simulink model "Model_TranslationEngine64"  (R2022b)
settings: Solver=FixedStepDiscrete  StartTime=0.0  StopTime=5  RelTol=1e-3  EnableMultiTasking=on
InitFcn:
  | % Initialize model
  | ModelSettings=BTConfig.GetModelSettings();
  | 
  | ModelSettings.Validate();
  | 
  | ModelInit;
  | 
  | 
  | % load library data
  | GainLibrary_data;
  | % Load saved values from partition process
  | CapturedConstMask.LoadMapFromFile(bdroot)
StartFcn:
  | % make sure all the simulated RTC requests are found
  | %RTC_SIM_OBJ.ValidateREQs();
undefined symbols (not defined in the file or in its folder): AA, BPLP, Column, NumHFRefBPF, NumHFRefLPF, NumMusicChannels, Row, VolumeMuteConfig
libraries: TuneVar x925, TOP x490, FeaturePath x111, CapturedConstLib x52
(part 29 of 34)

== system Model_TranslationEngine64/ModelPreAmp/DecRate/Medusa5H1/MedusaHoligram/Medusa5H1 Part 3/On/VLS Gains Computation/VLS Gains Pax/Fade Tuning/Foward Downmix Max ==
  TOP : TOP/TOP  TriggerInit=[440 20 585 80]  TopName=ForwardDownmixMax  DataTypeOut=single  BankNumber=0  PreOverlay=false  PostOverlay=false  Role=Automatic
      settings: SourceProductName=Bose Talaria
  TranslateTrigger : TuneVar/TranslateTrigger  TriggerInit=[286 -100 324 -45]
      settings: SourceProductName=Bose Talaria
  Trivial Translation : MATLAB Function  TreatAsAtomicUnit=on
  Tune Variable : TuneVar/TuneVar  TuneName=ForwardDownmixMax  SpecifyMaxSize=off  VariableDim=1 (Row)  MaxSize=[1 1]  TunabilityNumber=1  MinValue=[0]  MaxValue=[1]  TriggerInit=[-70 25 100 75]  MaskValue=tuneStruct.ForwardDownmixMax
      settings: SourceProductName=Bose Talaria
  wires:
  Tune Variable/1 -> Trivial Translation/1(ForwardDownmixMax)  "ForwardDownmixMax"
  Trivial Translation/1(TOP) -> TOP/1
  TranslateTrigger/1 -> Trivial Translation/Trigger

== system Model_TranslationEngine64/ModelPreAmp/DecRate/Medusa5H1/MedusaHoligram/Medusa5H1 Part 3/On/VLS Gains Computation/VLS Gains Pax/SLC Tuning/Detent Level ==
  TOP : TOP/TOP  TriggerInit=[405 22 635 78]  TopName=DetentLevel  DataTypeOut=single  BankNumber=0  PreOverlay=false  PostOverlay=false  Role=Automatic
      settings: SourceProductName=Bose Talaria
  TranslateTrigger : TuneVar/TranslateTrigger  TriggerInit=[266 -100 304 -45]
      settings: SourceProductName=Bose Talaria
  Trivial Translation : MATLAB Function  TreatAsAtomicUnit=on
  Tune Variable : TuneVar/TuneVar  TuneName=DetentLevel  SpecifyMaxSize=off  VariableDim=1 (Row)  MaxSize=[1 1]  TunabilityNumber=1  MinValue=[0]  MaxValue=[1]  TriggerInit=[-110 25 105 75]  MaskValue=tuneStruct.detentGain
      settings: SourceProductName=Bose Talaria
  wires:
  Tune Variable/1 -> Trivial Translation/1(detentGain)  "DetentLevel"
  Trivial Translation/1(TOP) -> TOP/1
  TranslateTrigger/1 -> Trivial Translation/Trigger

== system Model_TranslationEngine64/ModelPreAmp/DecRate/Medusa5H1/MedusaHoligram/Medusa5H1 Part 3/On/VLS Gains Computation/VLS Gains Pax/SLC Tuning/Interpolation Method ==
  TOP : TOP/TOP  TriggerInit=[440 20 585 80]  TopName=Interpolation_Method  DataTypeOut=single  BankNumber=0  PreOverlay=false  PostOverlay=false  Role=Automatic
      settings: SourceProductName=Bose Talaria
  TranslateTrigger : TuneVar/TranslateTrigger  TriggerInit=[306 -100 344 -45]
      settings: SourceProductName=Bose Talaria
  Trivial Translation : MATLAB Function  TreatAsAtomicUnit=on
  Tune Variable : TuneVar/TuneVar  TuneName=Interpolation_Method  SpecifyMaxSize=off  VariableDim=1 (Row)  MaxSize=[1 1]  TunabilityNumber=2  MinValue=[0]  MaxValue=[1]  TriggerInit=[-40 25 130 75]  MaskValue=tuneStruct.interpolationMethod
      settings: SourceProductName=Bose Talaria
  wires:
  Tune Variable/1 -> Trivial Translation/1(interpolationMethod)  "Interpolation_Method"
  Trivial Translation/1(TOP) -> TOP/1
  TranslateTrigger/1 -> Trivial Translation/Trigger

== system Model_TranslationEngine64/ModelPreAmp/DecRate/Medusa5H1/MedusaHoligram/Medusa5H1 Part 3/On/VLS Gains Computation/VLS Gains Pax/SLC Tuning/Max Level ==
  TOP : TOP/TOP  TriggerInit=[425 22 630 78]  TopName=MaxLevel  DataTypeOut=single  BankNumber=0  PreOverlay=false  PostOverlay=false  Role=Automatic
      settings: SourceProductName=Bose Talaria
  TranslateTrigger : TuneVar/TranslateTrigger  TriggerInit=[306 -100 344 -45]
      settings: SourceProductName=Bose Talaria
  Trivial Translation : MATLAB Function  TreatAsAtomicUnit=on
  Tune Variable : TuneVar/TuneVar  TuneName=MaxLevel  SpecifyMaxSize=off  VariableDim=1 (Row)  MaxSize=[1 1]  TunabilityNumber=1  MinValue=[0]  MaxValue=[1]  TriggerInit=[-55 25 145 75]  MaskValue=tuneStruct.maxGain
      settings: SourceProductName=Bose Talaria
  wires:
  Tune Variable/1 -> Trivial Translation/1(maxGain)  "MaxLevel"
  Trivial Translation/1(TOP) -> TOP/1
  TranslateTrigger/1 -> Trivial Translation/Trigger

== system Model_TranslationEngine64/ModelPreAmp/DecRate/Medusa5H1/MedusaHoligram/Medusa5H1 Part 3/On/VLS Gains Computation/VLS Gains Pax/SLC Tuning/Min Level ==
  TOP : TOP/TOP  TriggerInit=[360 17 565 73]  TopName=MinLevel  DataTypeOut=single  BankNumber=0  PreOverlay=false  PostOverlay=false  Role=Automatic
      settings: SourceProductName=Bose Talaria
  TranslateTrigger : TuneVar/TranslateTrigger  TriggerInit=[231 -105 269 -50]
      settings: SourceProductName=Bose Talaria
  Trivial Translation : MATLAB Function  TreatAsAtomicUnit=on
  Tune Variable : TuneVar/TuneVar  TuneName=MinLevel  SpecifyMaxSize=off  VariableDim=1 (Row)  MaxSize=[1 1]  TunabilityNumber=1  MinValue=[0]  MaxValue=[1]  TriggerInit=[-120 20 65 70]  MaskValue=tuneStruct.minGain
      settings: SourceProductName=Bose Talaria
  wires:
  Tune Variable/1 -> Trivial Translation/1(minGain)  "MinLevel"
  Trivial Translation/1(TOP) -> TOP/1
  TranslateTrigger/1 -> Trivial Translation/Trigger

== system Model_TranslationEngine64/ModelPreAmp/DecRate/AudioPilot35/Audiopilot_3_5/NoiseEstimationVariant/RegularNoiseEstimation/HFNoiseEstimatorCoh/PostProcessing/HfImpulseRejection/ComputeSmoothingFactor/MinstatAlphaFactor ==
  TOP : TOP/TOP  TriggerInit=[440 20 585 80]  TopName=MinstatAlphaFactor  DataTypeOut=single  BankNumber=BankNumber  PreOverlay=PreOverlay  PostOverlay=PostOverlay  Role=Automatic
      settings: SourceProductName=Bose Talaria
  TrivialTranslation : TuneVar/TrivialTranslation  TriggerInit=[300 28 350 72]
      settings: SourceProductName=Bose Talaria
  Tune Variable : TuneVar/TuneVar  TuneName=MinstatAlphaFactor  SpecifyMaxSize=off  VariableDim=1 (Row)  MaxSize=[1 1]  TunabilityNumber=1  MinValue=MinValue  MaxValue=MaxValue  TriggerInit=[20 25 190 75]  MaskValue=MaskValue
      settings: SourceProductName=Bose Talaria
  wires:
  TrivialTranslation/1 -> TOP/1
  Tune Variable/1 -> TrivialTranslation/1  "MinstatAlphaFactor"

== system Model_TranslationEngine64/ModelPreAmp/DecRate/AudioPilot35/Audiopilot_3_5/NoiseEstimationVariant/RegularNoiseEstimation/HFNoiseEstimatorCoh/PostProcessing/HfImpulseRejection/ComputeSmoothingFactor/MinstatAlphaMin ==
  TOP : TOP/TOP  TriggerInit=[440 20 585 80]  TopName=MinstatAlphaMin  DataTypeOut=single  BankNumber=BankNumber  PreOverlay=PreOverlay  PostOverlay=PostOverlay  Role=Automatic
      settings: SourceProductName=Bose Talaria
  TrivialTranslation : TuneVar/TrivialTranslation  TriggerInit=[300 28 350 72]
      settings: SourceProductName=Bose Talaria
  Tune Variable : TuneVar/TuneVar  TuneName=MinstatAlphaMin  SpecifyMaxSize=off  VariableDim=1 (Row)  MaxSize=[1 1]  TunabilityNumber=1  MinValue=MinValue  MaxValue=MaxValue  TriggerInit=[20 25 190 75]  MaskValue=MaskValue
      settings: SourceProductName=Bose Talaria
  wires:
  TrivialTranslation/1 -> TOP/1
  Tune Variable/1 -> TrivialTranslation/1  "MinstatAlphaMin"

== system Model_TranslationEngine64/ModelPreAmp/DecRate/AudioPilot35/Audiopilot_3_5/NoiseEstimationVariant/RegularNoiseEstimation/HFNoiseEstimatorCoh/PostProcessing/HfImpulseRejection/IntermediateCalculation1 /MinstatBeta ==
  TOP : TOP/TOP  TriggerInit=[440 20 585 80]  TopName=MinstatBeta  DataTypeOut=single  BankNumber=BankNumber  PreOverlay=PreOverlay  PostOverlay=PostOverlay  Role=Automatic
      settings: SourceProductName=Bose Talaria
  TrivialTranslation : TuneVar/TrivialTranslation  TriggerInit=[300 28 350 72]
      settings: SourceProductName=Bose Talaria
  Tune Variable : TuneVar/TuneVar  TuneName=MinstatBeta  SpecifyMaxSize=off  VariableDim=1 (Row)  MaxSize=[1 1]  TunabilityNumber=1  MinValue=MinValue  MaxValue=MaxValue  TriggerInit=[20 25 190 75]  MaskValue=MaskValue
      settings: SourceProductName=Bose Talaria
  wires:
  TrivialTranslation/1 -> TOP/1
  Tune Variable/1 -> TrivialTranslation/1  "MinstatBeta"

== system Model_TranslationEngine64/ModelPreAmp/DecRate/AudioPilot35/Audiopilot_3_5/NoiseEstimationVariant/RegularNoiseEstimation/HFNoiseEstimatorCoh/PostProcessing/HfImpulseRejection/IntermediateCalculation1 /MinstatMin ==
  TOP : TOP/TOP  TriggerInit=[440 20 585 80]  TopName=MinstatMin  DataTypeOut=single  BankNumber=BankNumber  PreOverlay=PreOverlay  PostOverlay=PostOverlay  Role=Automatic
      settings: SourceProductName=Bose Talaria
  TrivialTranslation : TuneVar/TrivialTranslation  TriggerInit=[300 28 350 72]
      settings: SourceProductName=Bose Talaria
  Tune Variable : TuneVar/TuneVar  TuneName=MinstatMin  SpecifyMaxSize=off  VariableDim=1 (Row)  MaxSize=[1 1]  TunabilityNumber=1  MinValue=MinValue  MaxValue=MaxValue  TriggerInit=[20 25 190 75]  MaskValue=MaskValue
      settings: SourceProductName=Bose Talaria
  wires:
  TrivialTranslation/1 -> TOP/1
  Tune Variable/1 -> TrivialTranslation/1  "MinstatMin"

== system Model_TranslationEngine64/ModelPreAmp/DecRate/AudioPilot35/Audiopilot_3_5/NoiseEstimationVariant/RegularNoiseEstimation/HFNoiseEstimatorCoh/PostProcessing/HfImpulseRejection/MinSearch/FlatnessHighIndex ==
  TOP : TOP/TOP  TriggerInit=[440 20 585 80]  TopName=FlatnessHighIndex  DataTypeOut=single  BankNumber=BankNumber  PreOverlay=PreOverlay  PostOverlay=PostOverlay  Role=Automatic
      settings: SourceProductName=Bose Talaria
  TrivialTranslation : TuneVar/TrivialTranslation  TriggerInit=[300 28 350 72]
      settings: SourceProductName=Bose Talaria
  Tune Variable : TuneVar/TuneVar  TuneName=FlatnessHighIndex  SpecifyMaxSize=off  VariableDim=1 (Row)  MaxSize=[1 1]  TunabilityNumber=1  MinValue=MinValue  MaxValue=MaxValue  TriggerInit=[20 25 190 75]  MaskValue=MaskValue
      settings: SourceProductName=Bose Talaria
  wires:
  TrivialTranslation/1 -> TOP/1
  Tune Variable/1 -> TrivialTranslation/1  "FlatnessHighIndex"

== system Model_TranslationEngine64/ModelPreAmp/DecRate/AudioPilot35/Audiopilot_3_5/NoiseEstimationVariant/RegularNoiseEstimation/HFNoiseEstimatorCoh/PostProcessing/HfImpulseRejection/MinSearch/FlatnessLowIndex ==
  TOP : TOP/TOP  TriggerInit=[440 20 585 80]  TopName=FlatnessLowIndex  DataTypeOut=single  BankNumber=BankNumber  PreOverlay=PreOverlay  PostOverlay=PostOverlay  Role=Automatic
      settings: SourceProductName=Bose Talaria
  TrivialTranslation : TuneVar/TrivialTranslation  TriggerInit=[300 28 350 72]
      settings: SourceProductName=Bose Talaria
  Tune Variable : TuneVar/TuneVar  TuneName=FlatnessLowIndex  SpecifyMaxSize=off  VariableDim=1 (Row)  MaxSize=[1 1]  TunabilityNumber=1  MinValue=MinValue  MaxValue=MaxValue  TriggerInit=[20 25 190 75]  MaskValue=MaskValue
      settings: SourceProductName=Bose Talaria
  wires:
  TrivialTranslation/1 -> TOP/1
  Tune Variable/1 -> TrivialTranslation/1  "FlatnessLowIndex"

== system Model_TranslationEngine64/ModelPreAmp/DecRate/AudioPilot35/Audiopilot_3_5/NoiseEstimationVariant/RegularNoiseEstimation/HFNoiseEstimatorCoh/PostProcessing/HfImpulseRejection/MinSearch/FlatnessThreshold ==
  TOP : TOP/TOP  TriggerInit=[440 20 585 80]  TopName=FlatnessThresh  DataTypeOut=single  BankNumber=BankNumber  PreOverlay=PreOverlay  PostOverlay=PostOverlay  Role=Automatic
      settings: SourceProductName=Bose Talaria
  TrivialTranslation : TuneVar/TrivialTranslation  TriggerInit=[300 28 350 72]
      settings: SourceProductName=Bose Talaria
  Tune Variable : TuneVar/TuneVar  TuneName=FlatnessThresh  SpecifyMaxSize=off  VariableDim=1 (Row)  MaxSize=[1 1]  TunabilityNumber=1  MinValue=MinValue  MaxValue=MaxValue  TriggerInit=[20 25 190 75]  MaskValue=MaskValue
      settings: SourceProductName=Bose Talaria
  wires:
  TrivialTranslation/1 -> TOP/1
  Tune Variable/1 -> TrivialTranslation/1  "FlatnessThresh"

== system Model_TranslationEngine64/ModelPreAmp/DecRate/AudioPilot35/Audiopilot_3_5/NoiseEstimationVariant/RegularNoiseEstimation/HFNoiseEstimatorCoh/PostProcessing/HfImpulseRejection/MinSearch/MinSearchCoef ==
  TOP : TOP/TOP  TriggerInit=[440 20 585 80]  TopName=MinSearchCoef  DataTypeOut=single  BankNumber=BankNumber  PreOverlay=PreOverlay  PostOverlay=PostOverlay  Role=Automatic
      settings: SourceProductName=Bose Talaria
  TrivialTranslation : TuneVar/TrivialTranslation  TriggerInit=[300 28 350 72]
      settings: SourceProductName=Bose Talaria
  Tune Variable : TuneVar/TuneVar  TuneName=MinSearchCoef  SpecifyMaxSize=off  VariableDim=1 (Row)  MaxSize=[1 1]  TunabilityNumber=1  MinValue=MinValue  MaxValue=MaxValue  TriggerInit=[20 25 190 75]  MaskValue=MaskValue
      settings: SourceProductName=Bose Talaria
  wires:
  TrivialTranslation/1 -> TOP/1
  Tune Variable/1 -> TrivialTranslation/1  "MinSearchCoef"

== system Model_TranslationEngine64/ModelPreAmp/DecRate/AudioPilot35/Audiopilot_3_5/NoiseEstimationVariant/RegularNoiseEstimation/HFNoiseEstimatorCoh/PostProcessing/HfImpulseRejection/MinSearch/MinSearchMinGain ==
  TOP : TOP/TOP  TriggerInit=[440 20 585 80]  TopName=MinSearchMinGain  DataTypeOut=single  BankNumber=BankNumber  PreOverlay=PreOverlay  PostOverlay=PostOverlay  Role=Automatic
      settings: SourceProductName=Bose Talaria
  TrivialTranslation : TuneVar/TrivialTranslation  TriggerInit=[300 28 350 72]
      settings: SourceProductName=Bose Talaria
  Tune Variable : TuneVar/TuneVar  TuneName=MinSearchMinGain  SpecifyMaxSize=off  VariableDim=1 (Row)  MaxSize=[1 1]  TunabilityNumber=1  MinValue=MinValue  MaxValue=MaxValue  TriggerInit=[20 25 190 75]  MaskValue=MaskValue
      settings: SourceProductName=Bose Talaria
  wires:
  TrivialTranslation/1 -> TOP/1
  Tune Variable/1 -> TrivialTranslation/1  "MinSearchMinGain"

== system Model_TranslationEngine64/ModelPreAmp/DecRate/AudioPilot35/Audiopilot_3_5/NoiseEstimationVariant/RegularNoiseEstimation/HFNoiseEstimatorCoh/PostProcessing/HfImpulseRejection/MinSearch/SubWinLen ==
  Sec2Samples : MATLAB Function  TreatAsAtomicUnit=on
  TOP : TOP/TOP  TriggerInit=[5 25 270 75]  TopName=SubWinLenSamples  DataTypeOut=single  BankNumber=0  PreOverlay=false  PostOverlay=false  Role=Automatic
      settings: SourceProductName=Bose Talaria
  TranslateTrigger : TuneVar/TranslateTrigger  TriggerInit=[-129 -100 -91 -45]
      settings: SourceProductName=Bose Talaria
  Tune Variable : TuneVar/TuneVar  TuneName=SubWinTimeS  SpecifyMaxSize=off  VariableDim=1 (Row)  MaxSize=[1 1]  TunabilityNumber=1  MinValue=[]  MaxValue=[]  TriggerInit=[-520 25 -255 75]  MaskValue=Config.ImpRejSubWindowTimeSec
      settings: SourceProductName=Bose Talaria
  wires:
  Tune Variable/1 -> Sec2Samples/1(time)  "SubWinTimeS"
  Sec2Samples/1(samples) -> TOP/1
  TranslateTrigger/1 -> Sec2Samples/Trigger

== system Model_TranslationEngine64/ModelPreAmp/DecRate/AudioPilot35/Audiopilot_3_5/NoiseEstimationVariant/RegularNoiseEstimation/HFNoiseEstimatorCoh/PostProcessing/HfImpulseRejection/SmoothingNoiseFloor/LevelUpdateCoef ==
  TOP : TOP/TOP  TriggerInit=[440 20 585 80]  TopName=LevelUpdateCoef  DataTypeOut=single  BankNumber=BankNumber  PreOverlay=PreOverlay  PostOverlay=PostOverlay  Role=Automatic
      settings: SourceProductName=Bose Talaria
  TrivialTranslation : TuneVar/TrivialTranslation  TriggerInit=[300 28 350 72]
      settings: SourceProductName=Bose Talaria
  Tune Variable : TuneVar/TuneVar  TuneName=LevelUpdateCoef  SpecifyMaxSize=off  VariableDim=1 (Row)  MaxSize=[1 1]  TunabilityNumber=1  MinValue=MinValue  MaxValue=MaxValue  TriggerInit=[20 25 190 75]  MaskValue=MaskValue
      settings: SourceProductName=Bose Talaria
  wires:
  TrivialTranslation/1 -> TOP/1
  Tune Variable/1 -> TrivialTranslation/1  "LevelUpdateCoef"

== system Model_TranslationEngine64/ModelPreAmp/DecRate/AudioPilot35/Audiopilot_3_5/NoiseEstimationVariant/RegularNoiseEstimation/HFNoiseEstimatorCoh/PreProcessing/Anti-Aliasing Filter/InnerLink/PoolIirTunableWithReset ==
  CapturedTuneConst : CapturedConstLib/CapturedConst  TriggerInit=[-600 302 -500 338]  Role=Automatic
      settings: SourceProductName=Bose Talaria
  FeaturePath : FeaturePath/FeaturePath  FeatureName=PreprocessAntiAlias  IsGroup=off  GroupNumber=-1  IsModule=off  TriggerInit=[-750 -81 -635 26]
      settings: SourceProductName=Bose Talaria
  TOP : TOP/TOP  TriggerInit=[-145 187 5 243]  TopName=PooliirNumStages  DataTypeOut=uint32  BankNumber=0  PreOverlay=false  PostOverlay=Config.VariantObj.PostOverlayRequired  Role=Automatic
      settings: SourceProductName=Bose Talaria
  TOP1 : TOP/TOP  TriggerInit=[-140 277 10 333]  TopName=pooliirCoeffs  DataTypeOut=single  BankNumber=0  PreOverlay=false  PostOverlay=Config.VariantObj.PostOverlayRequired  Role=Automatic
      settings: SourceProductName=Bose Talaria
  TranslateTrigger : TuneVar/TranslateTrigger  TriggerInit=[-339 35 -301 90]
      settings: SourceProductName=Bose Talaria
  Translation : MATLAB Function  TreatAsAtomicUnit=on  mask{MaxNumStages=Config.MaxNumStages, VariantUint8=Config.Variant.Uint8Str}
      mask prompts: VariantUint8 "Variant"
  Tune Variable1 : TuneVar/TuneVar  TuneName=numStages  SpecifyMaxSize=off  VariableDim=1 (Row)  MaxSize=[1 1]  TunabilityNumber=1  MinValue=[]  MaxValue=[]  TriggerInit=[-750 235 -580 285]  MaskValue=Config.TuneDefaults.NumStages
      settings: SourceProductName=Bose Talaria
  Tune Variable2 : TuneVar/TuneVar  TuneName=sosCoefficients  SpecifyMaxSize=on  VariableDim=1 (Row)  MaxSize=[Config.MaxNumStages 6]  TunabilityNumber=1  MinValue=[]  MaxValue=[]  TriggerInit=[-750 175 -580 225]  MaskValue=Config.TuneDefaults.SosCoefficients
      settings: SourceProductName=Bose Talaria
  wires:
  TranslateTrigger/1 -> Translation/Trigger
  Tune Variable2/1 -> Translation/1(RawSOS)  "sosCoefficients"
  Translation/2(PoolCoeffs) -> TOP1/1
  Translation/1(PoolNumStages) -> TOP/1
  Tune Variable1/1 -> Translation/2(NumStages)  "numStages"
  CapturedTuneConst/1 -> Translation/3(NumChannels)

== system Model_TranslationEngine64/ModelPreAmp/DecRate/AudioPilot35/Audiopilot_3_5/NoiseEstimationVariant/RegularNoiseEstimation/HFNoiseEstimatorCoh/PreProcessing/Bandpass or Lowpass Filter/InnerLink/PoolIirTunableWithReset ==
  CapturedTuneConst : CapturedConstLib/CapturedConst  TriggerInit=[-600 302 -500 338]  Role=Automatic
      settings: SourceProductName=Bose Talaria
  FeaturePath : FeaturePath/FeaturePath  FeatureName=PreprocessBandpassLowpass  IsGroup=off  GroupNumber=-1  IsModule=off  TriggerInit=[-750 -81 -635 26]
      settings: SourceProductName=Bose Talaria
  TOP : TOP/TOP  TriggerInit=[-145 187 5 243]  TopName=PooliirNumStages  DataTypeOut=uint32  BankNumber=0  PreOverlay=false  PostOverlay=Config.VariantObj.PostOverlayRequired  Role=Automatic
      settings: SourceProductName=Bose Talaria
  TOP1 : TOP/TOP  TriggerInit=[-140 277 10 333]  TopName=pooliirCoeffs  DataTypeOut=single  BankNumber=0  PreOverlay=false  PostOverlay=Config.VariantObj.PostOverlayRequired  Role=Automatic
      settings: SourceProductName=Bose Talaria
  TranslateTrigger : TuneVar/TranslateTrigger  TriggerInit=[-339 35 -301 90]
      settings: SourceProductName=Bose Talaria
  Translation : MATLAB Function  TreatAsAtomicUnit=on  mask{MaxNumStages=Config.MaxNumStages, VariantUint8=Config.Variant.Uint8Str}
      mask prompts: VariantUint8 "Variant"
  Tune Variable1 : TuneVar/TuneVar  TuneName=numStages  SpecifyMaxSize=off  VariableDim=1 (Row)  MaxSize=[1 1]  TunabilityNumber=1  MinValue=[]  MaxValue=[]  TriggerInit=[-750 235 -580 285]  MaskValue=Config.TuneDefaults.NumStages
      settings: SourceProductName=Bose Talaria
  Tune Variable2 : TuneVar/TuneVar  TuneName=sosCoefficients  SpecifyMaxSize=on  VariableDim=1 (Row)  MaxSize=[Config.MaxNumStages 6]  TunabilityNumber=1  MinValue=[]  MaxValue=[]  TriggerInit=[-750 175 -580 225]  MaskValue=Config.TuneDefaults.SosCoefficients
      settings: SourceProductName=Bose Talaria
  wires:
  TranslateTrigger/1 -> Translation/Trigger
  Tune Variable2/1 -> Translation/1(RawSOS)  "sosCoefficients"
  Translation/2(PoolCoeffs) -> TOP1/1
  Translation/1(PoolNumStages) -> TOP/1
  Tune Variable1/1 -> Translation/2(NumStages)  "numStages"
  CapturedTuneConst/1 -> Translation/3(NumChannels)

== system Model_TranslationEngine64/ModelPreAmp/DecRate/AudioPilot35/Audiopilot_3_5/NoiseEstimationVariant/RegularNoiseEstimation/LFNoiseEstimatorCoh/LfPreProcess/FilterMic/InnerLink/PoolIirTunableWithReset ==
  CapturedTuneConst : CapturedConstLib/CapturedConst  TriggerInit=[-600 302 -500 338]  Role=Automatic
      settings: SourceProductName=Bose Talaria
  FeaturePath : FeaturePath/FeaturePath  FeatureName=Mic  IsGroup=off  GroupNumber=-1  IsModule=off  TriggerInit=[-750 -81 -635 26]
      settings: SourceProductName=Bose Talaria
  TOP : TOP/TOP  TriggerInit=[-145 187 5 243]  TopName=PooliirNumStages  DataTypeOut=uint32  BankNumber=0  PreOverlay=false  PostOverlay=Config.VariantObj.PostOverlayRequired  Role=Automatic
      settings: SourceProductName=Bose Talaria
  TOP1 : TOP/TOP  TriggerInit=[-140 277 10 333]  TopName=pooliirCoeffs  DataTypeOut=single  BankNumber=0  PreOverlay=false  PostOverlay=Config.VariantObj.PostOverlayRequired  Role=Automatic
      settings: SourceProductName=Bose Talaria
  TranslateTrigger : TuneVar/TranslateTrigger  TriggerInit=[-339 35 -301 90]
      settings: SourceProductName=Bose Talaria
  Translation : MATLAB Function  TreatAsAtomicUnit=on  mask{MaxNumStages=Config.MaxNumStages, VariantUint8=Config.Variant.Uint8Str}
      mask prompts: VariantUint8 "Variant"
  Tune Variable1 : TuneVar/TuneVar  TuneName=numStages  SpecifyMaxSize=off  VariableDim=1 (Row)  MaxSize=[1 1]  TunabilityNumber=1  MinValue=[]  MaxValue=[]  TriggerInit=[-750 235 -580 285]  MaskValue=Config.TuneDefaults.NumStages
      settings: SourceProductName=Bose Talaria
  Tune Variable2 : TuneVar/TuneVar  TuneName=sosCoefficients  SpecifyMaxSize=on  VariableDim=1 (Row)  MaxSize=[Config.MaxNumStages 6]  TunabilityNumber=1  MinValue=[]  MaxValue=[]  TriggerInit=[-750 175 -580 225]  MaskValue=Config.TuneDefaults.SosCoefficients
      settings: SourceProductName=Bose Talaria
  wires:
  TranslateTrigger/1 -> Translation/Trigger
  Tune Variable2/1 -> Translation/1(RawSOS)  "sosCoefficients"
  Translation/2(PoolCoeffs) -> TOP1/1
  Translation/1(PoolNumStages) -> TOP/1
  Tune Variable1/1 -> Translation/2(NumStages)  "numStages"
  CapturedTuneConst/1 -> Translation/3(NumChannels)

== system Model_TranslationEngine64/ModelPreAmp/DecRate/AudioPilot35/Audiopilot_3_5/NoiseEstimationVariant/RegularNoiseEstimation/LFNoiseEstimatorCoh/LfPreProcess/FilterRef/InnerLink/PoolIirTunableWithReset ==
  CapturedTuneConst : CapturedConstLib/CapturedConst  TriggerInit=[-600 302 -500 338]  Role=Automatic
      settings: SourceProductName=Bose Talaria
  FeaturePath : FeaturePath/FeaturePath  FeatureName=Ref  IsGroup=off  GroupNumber=-1  IsModule=off  TriggerInit=[-750 -81 -635 26]
      settings: SourceProductName=Bose Talaria
  TOP : TOP/TOP  TriggerInit=[-145 187 5 243]  TopName=PooliirNumStages  DataTypeOut=uint32  BankNumber=0  PreOverlay=false  PostOverlay=Config.VariantObj.PostOverlayRequired  Role=Automatic
      settings: SourceProductName=Bose Talaria
  TOP1 : TOP/TOP  TriggerInit=[-140 277 10 333]  TopName=pooliirCoeffs  DataTypeOut=single  BankNumber=0  PreOverlay=false  PostOverlay=Config.VariantObj.PostOverlayRequired  Role=Automatic
      settings: SourceProductName=Bose Talaria
  TranslateTrigger : TuneVar/TranslateTrigger  TriggerInit=[-339 35 -301 90]
      settings: SourceProductName=Bose Talaria
  Translation : MATLAB Function  TreatAsAtomicUnit=on  mask{MaxNumStages=Config.MaxNumStages, VariantUint8=Config.Variant.Uint8Str}
      mask prompts: VariantUint8 "Variant"
  Tune Variable1 : TuneVar/TuneVar  TuneName=numStages  SpecifyMaxSize=off  VariableDim=1 (Row)  MaxSize=[1 1]  TunabilityNumber=1  MinValue=[]  MaxValue=[]  TriggerInit=[-750 235 -580 285]  MaskValue=Config.TuneDefaults.NumStages
      settings: SourceProductName=Bose Talaria
  Tune Variable2 : TuneVar/TuneVar  TuneName=sosCoefficients  SpecifyMaxSize=on  VariableDim=1 (Row)  MaxSize=[Config.MaxNumStages 6]  TunabilityNumber=1  MinValue=[]  MaxValue=[]  TriggerInit=[-750 175 -580 225]  MaskValue=Config.TuneDefaults.SosCoefficients
      settings: SourceProductName=Bose Talaria
  wires:
  TranslateTrigger/1 -> Translation/Trigger
  Tune Variable2/1 -> Translation/1(RawSOS)  "sosCoefficients"
  Translation/2(PoolCoeffs) -> TOP1/1
  Translation/1(PoolNumStages) -> TOP/1
  Tune Variable1/1 -> Translation/2(NumStages)  "numStages"
  CapturedTuneConst/1 -> Translation/3(NumChannels)

== system Model_TranslationEngine64/ModelPreAmp/DecRate/Medusa5H1/MedusaHoligram/Medusa5H1 Part 2/Decimated-Rate FDP/Fdp/FreqDomainProcessing/CalculateAndApplyCoefficients/DeciRate/Calculate coefficients ==
  note: Rate Transition blocks are inserted after TOPs to convert their sample rate
      | to decimated rate. Initially their sample rate is inherited from the fastest one
      | of all the blocks that use it, which happen to be either inside full-rate block,
      | or the fastest sample rate in the model.
  FeaturePath : FeaturePath/FeaturePath  FeatureName=Coeffs  IsGroup=off  GroupNumber=-1  IsModule=off  TriggerInit=[-545 -1 -430 106]
      settings: SourceProductName=Bose Talaria
  StretchParamsTuning : Subsystem

== system Model_TranslationEngine64/ModelPreAmp/DecRate/Medusa5H1/MedusaHoligram/Medusa5H1 Part 2/Full-Rate FDP/Fdp/FreqDomainProcessing/CalculateAndApplyCoefficients/FullRate/Calculate coefficients ==
  FeaturePath : FeaturePath/FeaturePath  FeatureName=Coeffs  IsGroup=off  GroupNumber=-1  IsModule=off  TriggerInit=[1075 99 1190 206]
      settings: SourceProductName=Bose Talaria
  StretchParams : Subsystem

== system Model_TranslationEngine64/ModelPreAmp/DecRate/Medusa5H1/MedusaHoligram/Medusa5H1 Part 2/Decimated-Rate FDP/Fdp/FreqDomainProcessing/CalculateAndApplyCoefficients/DeciRate/Calculate coefficients/StretchParamsTuning ==
  TOP : TOP/TOP  TriggerInit=[1190 -388 1425 -332]  TopName=XpMax  DataTypeOut=single  BankNumber=0  PreOverlay=false  PostOverlay=false  Role=Automatic
      settings: SourceProductName=Bose Talaria
  TOP1 : TOP/TOP  TriggerInit=[1190 -310 1425 -250]  TopName=LokRokMaxScaleFactor  DataTypeOut=single  BankNumber=0  PreOverlay=false  PostOverlay=false  Role=Automatic
      settings: SourceProductName=Bose Talaria
  TOP2 : TOP/TOP  TriggerInit=[1195 -83 1430 -17]  TopName=ESDUpperbounddB  DataTypeOut=single  BankNumber=0  PreOverlay=false  PostOverlay=false  Role=Automatic
      settings: SourceProductName=Bose Talaria
  TOP3 : TOP/TOP  TriggerInit=[1195 0 1430 60]  TopName=ESDLowerbounddB  DataTypeOut=single  BankNumber=0  PreOverlay=false  PostOverlay=false  Role=Automatic
      settings: SourceProductName=Bose Talaria
  TOP4 : TOP/TOP  TriggerInit=[1195 80 1430 140]  TopName=ESDStepSize  DataTypeOut=single  BankNumber=0  PreOverlay=false  PostOverlay=false  Role=Automatic
      settings: SourceProductName=Bose Talaria
  TOP5 : TOP/TOP  TriggerInit=[1190 -230 1425 -170]  TopName=XpMin  DataTypeOut=single  BankNumber=0  PreOverlay=false  PostOverlay=false  Role=Automatic
      settings: SourceProductName=Bose Talaria
  TranslateTrigger : TuneVar/TranslateTrigger  TriggerInit=[1036 -460 1074 -425]
      settings: SourceProductName=Bose Talaria
  TranslateTrigger3 : TuneVar/TranslateTrigger  TriggerInit=[1041 -145 1079 -110]
      settings: SourceProductName=Bose Talaria
  Trivial Translation : MATLAB Function  TreatAsAtomicUnit=on
  Trivial Translation3 : MATLAB Function  TreatAsAtomicUnit=on
  Tune Variable1 : TuneVar/TuneVar  Description=Upper threshold on Excessive Stretch Detector (ESD) metric.  TuneName=ESDUpperbounddB  SpecifyMaxSize=off  VariableDim=1 (Row)  MaxSize=[1 1]  TunabilityNumber=1  MinValue=[]  MaxValue=[]  TriggerInit=[20 425 245 475]  MaskValue=Config.TuneDefaults.FdpCoeffsESDUpperbounddB
      settings: SourceProductName=Bose Talaria
  Tune Variable2 : TuneVar/TuneVar  Description=Lower threshold on Excessive Stretch Detector (ESD) metric.  TuneName=ESDLowerbounddB  SpecifyMaxSize=off  VariableDim=1 (Row)  MaxSize=[1 1]  TunabilityNumber=1  MinValue=[]  MaxValue=[]  TriggerInit=[20 545 240 595]  MaskValue=Config.TuneDefaults.FdpCoeffsDeciRateESDLowerbounddB
      settings: SourceProductName=Bose Talaria
  Tune Variable3 : TuneVar/TuneVar  Description=Minimum stretch factor - must be in range [0,1).  TuneName=XpMin  SpecifyMaxSize=off  VariableDim=1 (Row)  MaxSize=[1 1]  TunabilityNumber=1  MinValue=0  MaxValue=1  TriggerInit=[45 235 215 285]  MaskValue=Config.TuneDefaults.FdpCoeffsXpMin
      settings: SourceProductName=Bose Talaria
  wires:
  Tune Variable1/1 -> Trivial Translation3/1(ESDUpperbounddBIn)  "ESDUpperbounddB"
  Trivial Translation3/1(ESDUpperbounddB) -> TOP2/1
  TranslateTrigger/1 -> Trivial Translation/Trigger
  TranslateTrigger3/1 -> Trivial Translation3/Trigger
  Trivial Translation/3(XpMin) -> TOP5/1
  Trivial Translation3/2(ESDLowerbounddB) -> TOP3/1
  Trivial Translation/1(XpMax) -> TOP/1
  Tune Variable3/1 -> Trivial Translation/2(XpMinIn)  "XpMin"
  Trivial Translation/2(LokRokMaxScaleFactor) -> TOP1/1
  [deciRateXpMax] -> Trivial Translation/1(XpMaxIn)  "XpMax"
  Trivial Translation3/3(ESDStepSize) -> TOP4/1
  Tune Variable2/1 -> Trivial Translation3/2(ESDLowerbounddBIn)  "ESDLowerbounddB"

== system Model_TranslationEngine64/ModelPreAmp/DecRate/Medusa5H1/MedusaHoligram/Medusa5H1 Part 2/Full-Rate FDP/Fdp/FreqDomainProcessing/CalculateAndApplyCoefficients/FullRate/Calculate coefficients/StretchParams ==
  TOP : TOP/TOP  TriggerInit=[970 -388 1200 -332]  TopName=XpMax  DataTypeOut=single  BankNumber=0  PreOverlay=false  PostOverlay=false  Role=Automatic
      settings: SourceProductName=Bose Talaria
  TOP1 : TOP/TOP  TriggerInit=[970 -310 1205 -250]  TopName=LokRokMaxScaleFactor  DataTypeOut=single  BankNumber=0  PreOverlay=false  PostOverlay=false  Role=Automatic
      settings: SourceProductName=Bose Talaria
  TOP2 : TOP/TOP  TriggerInit=[970 -78 1205 -12]  TopName=ESDUpperbounddB  DataTypeOut=single  BankNumber=0  PreOverlay=false  PostOverlay=false  Role=Automatic
      settings: SourceProductName=Bose Talaria
  TOP3 : TOP/TOP  TriggerInit=[970 5 1205 65]  TopName=ESDLowerbounddB  DataTypeOut=single  BankNumber=0  PreOverlay=false  PostOverlay=false  Role=Automatic
      settings: SourceProductName=Bose Talaria
  TOP4 : TOP/TOP  TriggerInit=[970 85 1205 145]  TopName=ESDStepSize  DataTypeOut=single  BankNumber=0  PreOverlay=false  PostOverlay=false  Role=Automatic
      settings: SourceProductName=Bose Talaria
  TOP5 : TOP/TOP  TriggerInit=[970 -230 1205 -170]  TopName=XpMin  DataTypeOut=single  BankNumber=0  PreOverlay=false  PostOverlay=false  Role=Automatic
      settings: SourceProductName=Bose Talaria
  TranslateTrigger : TuneVar/TranslateTrigger  TriggerInit=[816 -460 854 -425]
      settings: SourceProductName=Bose Talaria
  TranslateTrigger3 : TuneVar/TranslateTrigger  TriggerInit=[816 -140 854 -105]
      settings: SourceProductName=Bose Talaria
  Trivial Translation : MATLAB Function  TreatAsAtomicUnit=on
  Trivial Translation3 : MATLAB Function  TreatAsAtomicUnit=on
  Tune Variable : TuneVar/TuneVar  Description=Maximum stretch factor - must be in range [0,1).  TuneName=XpMax  SpecifyMaxSize=off  VariableDim=1 (Row)  MaxSize=[1 1]  TunabilityNumber=1  MinValue=0  MaxValue=1  TriggerInit=[45 95 215 145]  MaskValue=Config.TuneDefaults.FdpFullRateXpMax
      settings: SourceProductName=Bose Talaria
  Tune Variable1 : TuneVar/TuneVar  Description=Upper threshold on Excessive Stretch Detector (ESD) metric.  TuneName=ESDUpperbounddB  SpecifyMaxSize=off  VariableDim=1 (Row)  MaxSize=[1 1]  TunabilityNumber=1  MinValue=[]  MaxValue=[]  TriggerInit=[20 430 235 480]  MaskValue=Config.TuneDefaults.FdpCoeffsESDUpperbounddB
      settings: SourceProductName=Bose Talaria
  Tune Variable2 : TuneVar/TuneVar  Description=Lower threshold on Excessive Stretch Detector (ESD) metric.  TuneName=ESDLowerbounddB  SpecifyMaxSize=off  VariableDim=1 (Row)  MaxSize=[1 1]  TunabilityNumber=1  MinValue=[]  MaxValue=[]  TriggerInit=[20 550 235 600]  MaskValue=Config.TuneDefaults.FdpCoeffsFullRateESDLowerbounddB
      settings: SourceProductName=Bose Talaria
  Tune Variable3 : TuneVar/TuneVar  Description=Minimum stretch factor - must be in range [0,1)  TuneName=XpMin  SpecifyMaxSize=off  VariableDim=1 (Row)  MaxSize=[1 1]  TunabilityNumber=1  MinValue=0  MaxValue=1  TriggerInit=[45 175 215 225]  MaskValue=Config.TuneDefaults.FdpCoeffsXpMin
      settings: SourceProductName=Bose Talaria
  wires:
  Tune Variable3/1 -> Trivial Translation/2(XpMinIn)  "XpMin"
  [deciRateXpMax] -> Trivial Translation/3(deciXpMaxIn)  "XpMax"
  Trivial Translation/1(XpMax) -> TOP/1
  Tune Variable2/1 -> Trivial Translation3/2(ESDLowerbounddBIn)  "ESDLowerbounddB"
  Tune Variable/1 -> Trivial Translation/1(XpMaxIn)  "XpMax"
  Trivial Translation3/2(ESDLowerbounddB) -> TOP3/1
  TranslateTrigger/1 -> Trivial Translation/Trigger
  Trivial Translation3/1(ESDUpperbounddB) -> TOP2/1
  Trivial Translation3/3(ESDStepSize) -> TOP4/1
  Trivial Translation/3(XpMin) -> TOP5/1
  TranslateTrigger3/1 -> Trivial Translation3/Trigger
  Trivial Translation/2(LokRokMaxScaleFactor) -> TOP1/1
  Tune Variable1/1 -> Trivial Translation3/1(ESDUpperbounddBIn)  "ESDUpperbounddB"

== matlab function Model_TranslationEngine64/ModelPreAmp/DecRate/Medusa5H1/MedusaHoligram/Medusa5H1 Part 3/On/VLS Gains Computation/VLS Gains Drv/SLC Tuning/Interpolation Method/Trivial Translation ==
  data: TOP output; interpolationMethod input
  events: trigger input FUNCTION_CALL_EVENT
function TOP  = fcn(interpolationMethod)
%#codegen
% Checks if the parameter satisfies dimensionality requirements
if(numel(interpolationMethod.Value) ~= 1)
   TranslateError('The parameter ''medusa_surround_db_interpolation'' must be single dimensional.'); 
end

% Checks if the parameter value follows bound requirements
if((interpolationMethod.Value ~= 0) && (interpolationMethod.Value ~= 1))
   TranslateError('The value of ''medusa_surround_db_interpolation'' must be either 0 (for linear interpolation) or 1 (for dB-linear interpolation).'); 
end

TOP = interpolationMethod.Value;

end

== matlab function Model_TranslationEngine64/ModelPreAmp/DecRate/AudioPilot35/EntertainmentLevelDetection/AudiopilotLevelDetect/AudiopilotLevelDetect/FastDecay/sec2samples ==
  data: y output; u input; FrameRate parameter
  events: trigger input FUNCTION_CALL_EVENT
function y  = fcn(u,FrameRate)
%#codegen

y = -abs(u.Value/FrameRate);

== matlab function Model_TranslationEngine64/ModelPreAmp/DecRate/Medusa5H1/MedusaHoligram/Medusa5H1 Part 3/On/VLS Gains Computation/VLS Gains Drv/SLC Tuning/Max Level/Trivial Translation ==
  data: TOP output; maxGain input; configStruct parameter
  events: trigger input FUNCTION_CALL_EVENT
function TOP  = fcn(maxGain, configStruct)
%#codegen

% Checks if the parameter satisfies dimensionality requirements
if(maxGain.Size(1) ~= configStruct.numGains)
    TranslateError('The parameter ''VLS_gains_max'' must be a %d element vector.', configStruct.numGains);
end

% Checks if the parameter values follow bound requirements
checkValues = (maxGain.Value < 0);
if(sum(sum(checkValues)))          % Results in 0 if all values in the matrix respect the bound requirements
    TranslateError('The weights in ''VLS_gains_max'' must be greater than or equal to 0.');
end

TOP = maxGain.Value;

end

== matlab function Model_TranslationEngine64/ModelPreAmp/DecRate/Medusa5H1/MedusaHoligram/Medusa5H1 Part 3/On/VLS Gains Computation/VLS Gains Drv/SLC Tuning/Min Level/Trivial Translation ==
  data: TOP output; minGain input; configStruct parameter
  events: trigger input FUNCTION_CALL_EVENT
function TOP  = fcn(minGain, configStruct)
%#codegen

% Checks if the parameter satisfies dimensionality requirements
if(minGain.Size(1) ~= configStruct.numGains)
    TranslateError('The parameter ''VLS_gains_min'' must be a %d element vector.', configStruct.numGains);
end

% Checks if the parameter values follow bound requirements
checkValues = (minGain.Value < 0);
if(sum(sum(checkValues)))          % Results in 0 if all values in the matrix respect the bound requirements
    TranslateError('The weights in ''VLS_gains_min'' must be greater than or equal to 0.');
end

TOP = minGain.Value;

end

== matlab function Model_TranslationEngine64/ModelPreAmp/DecRate/Medusa5H1/MedusaHoligram/Medusa5H1 Part 3/On/VLS Gains Computation/VLS Gains Pax/Fade Tuning/Forward Downmix Threshold/Trivial Translation ==
  data: TOP output; ForwardDownmixThreshold input
  events: trigger input FUNCTION_CALL_EVENT
function TOP  = fcn(ForwardDownmixThreshold)
%#codegen
% Checks if the parameter satisfies dimensionality requirements
if(numel(ForwardDownmixThreshold.Value) ~= 1)
   TranslateError('The parameter ''medusa_forward_downmix_threshold'' must be single dimensional.'); 
end

% Checks if the parameter value follows bound requirements
if((ForwardDownmixThreshold.Value < 0) || (ForwardDownmixThreshold.Value > 1))
   TranslateError('The value of ''medusa_forward_downmix_threshold'' must be between 0 and 1.'); 
end

TOP = ForwardDownmixThreshold.Value;

end

== matlab function Model_TranslationEngine64/ModelPreAmp/DecRate/Medusa5H1/MedusaHoligram/Medusa5H1 Part 3/On/VLS Gains Computation/VLS Gains Pax/Fade Tuning/Foward Downmix Max/Trivial Translation ==
  data: TOP output; ForwardDownmixMax input
  events: trigger input FUNCTION_CALL_EVENT
function TOP  = fcn(ForwardDownmixMax)
%#codegen
% Checks if the parameter satisfies dimensionality requirements
if(numel(ForwardDownmixMax.Value) ~= 1)
   TranslateError('The parameter ''medusa_forward_downmix_max'' must be single dimensional.'); 
end

% Checks if the parameter value follows bound requirements
if((ForwardDownmixMax.Value < 0) || (ForwardDownmixMax.Value > 1))
   TranslateError('The value of ''medusa_forward_downmix_max'' must be between 0 and 1.'); 
end

TOP = ForwardDownmixMax.Value;

end

== matlab function Model_TranslationEngine64/ModelPreAmp/DecRate/Medusa5H1/MedusaHoligram/Medusa5H1 Part 4/On/FR IIR Holigram EQ/IIR/PoolIirTunableWithReset/Translation ==
  data: RawSOS input; NumStages input; PoolNumStages output; PoolCoeffs output; MaxNumStages parameter; VariantUint8 parameter; NumChannels input
  events: trigger input FUNCTION_CALL_EVENT
function [PoolNumStages, PoolCoeffs] = pooliirTranslation(RawSOS, NumStages, MaxNumStages, VariantUint8,  NumChannels)
%#codegen

% Translation from raw SOS for pool SOS

% Some build time sanity size checking before calling the translation
if numel(NumStages.Value) ~= NumChannels
    error('Size of num stages has to match number of input channels')
end

if RawSOS.Size(2) ~= 6
    error ('Coefficient pool matrix must have 6 columns')
end

[PoolNumStages, PoolCoeffs] = poolIirTranslation(RawSOS, NumStages, MaxNumStages, VariantUint8);

% VariantStr = char(VariantUint8);
% switch (VariantStr)
%     case {"Generic","SharcPlusCore"}
%         % These variants order biquad coefficients in a compacted form
%         [PoolNumStages, PoolCoeffs] = pooliirTranslationFcn(RawSOS, NumStages, MaxNumStages);
%     case {"SharcPlusAccelGul","SharcPlusAccelGxp"}
%         % These variants order biquad coefficients for the ADI accelerator
%         [PoolNumStages, PoolCoeffs] = pooliirAccelTranslationFcn(RawSOS, NumStages, MaxNumStages);
%     case{"Hexagon"}
%         % Hexagon specific order for biquad coefficients 
%         [PoolNumStages, PoolCoeffs] = PoolIirHexagonTranslationFcn(RawSOS, NumStages, MaxNumStages);
%     case{"ArmNeonV7V8"}
%         [PoolNumStages, PoolCoeffs] = PoolIirArmNeonV7V8TranslationFcn(RawSOS, NumStages, MaxNumStages);
%     otherwise
%         % This is a build-time error, not a translation error. The
%         % selected build-time variant is not supported for translation
%         error('Invalid implementation type: [%s]', VariantStr);
% end

end

== matlab function Model_TranslationEngine64/ModelPreAmp/DecRate/Medusa5H1/MedusaHoligram/Medusa5H1 Part 4/On/DR Mix Matrix with Hybrid Holigram EQ/Tune Translations/translation ==
  data: FIRCoeffs output; FIRCoeffsIn input; FIRLengths output; FIRLengthsIn input; PaddedFIRLengthsIn input; PaddedFIRLengths output
  events: trigger input FUNCTION_CALL_EVENT
function [FIRCoeffs, FIRLengths, PaddedFIRLengths] = fcn(FIRCoeffsIn, FIRLengthsIn, PaddedFIRLengthsIn)

FIRCoeffs = FIRCoeffsIn.Value;
FIRLengths = FIRLengthsIn.Value;
PaddedFIRLengths = PaddedFIRLengthsIn.Value;

== matlab function Model_TranslationEngine64/ModelPreAmp/DecRate/Medusa5H1/MedusaHoligram/Medusa5H1 Part 4/On/Headrest Comp EQ/IIR/PoolIirTunableWithReset/Translation ==
  data: RawSOS input; NumStages input; PoolNumStages output; PoolCoeffs output; MaxNumStages parameter; VariantUint8 parameter; NumChannels input
  events: trigger input FUNCTION_CALL_EVENT
function [PoolNumStages, PoolCoeffs] = pooliirTranslation(RawSOS, NumStages, MaxNumStages, VariantUint8,  NumChannels)
%#codegen

% Translation from raw SOS for pool SOS

% Some build time sanity size checking before calling the translation
if numel(NumStages.Value) ~= NumChannels
    error('Size of num stages has to match number of input channels')
end

if RawSOS.Size(2) ~= 6
    error ('Coefficient pool matrix must have 6 columns')
end

[PoolNumStages, PoolCoeffs] = poolIirTranslation(RawSOS, NumStages, MaxNumStages, VariantUint8);

% VariantStr = char(VariantUint8);
% switch (VariantStr)
%     case {"Generic","SharcPlusCore"}
%         % These variants order biquad coefficients in a compacted form
%         [PoolNumStages, PoolCoeffs] = pooliirTranslationFcn(RawSOS, NumStages, MaxNumStages);
%     case {"SharcPlusAccelGul","SharcPlusAccelGxp"}
%         % These variants order biquad coefficients for the ADI accelerator
%         [PoolNumStages, PoolCoeffs] = pooliirAccelTranslationFcn(RawSOS, NumStages, MaxNumStages);
%     case{"Hexagon"}
%         % Hexagon specific order for biquad coefficients 
%         [PoolNumStages, PoolCoeffs] = PoolIirHexagonTranslationFcn(RawSOS, NumStages, MaxNumStages);
%     case{"ArmNeonV7V8"}
%         [PoolNumStages, PoolCoeffs] = PoolIirArmNeonV7V8TranslationFcn(RawSOS, NumStages, MaxNumStages);
%     otherwise
%         % This is a build-time error, not a translation error. The
%         % selected build-time variant is not supported for translation
%         error('Invalid implementation type: [%s]', VariantStr);
% end

end

== matlab function Model_TranslationEngine64/ModelPreAmp/DecRate/Medusa5H1/MedusaHoligram/Medusa5H1 Part 4/On/Headrest Comp EQ/translation ==
  data: FIRCoeffs output; FIRCoeffsIn input; FIRLengths output; FIRLengthsIn input; PaddedFIRLengthsIn input; PaddedFIRLengths output
  events: trigger input FUNCTION_CALL_EVENT
function [FIRCoeffs, FIRLengths, PaddedFIRLengths] = fcn(FIRCoeffsIn, FIRLengthsIn, PaddedFIRLengthsIn)

FIRCoeffs = FIRCoeffsIn.Value;
FIRLengths = FIRLengthsIn.Value;
PaddedFIRLengths = PaddedFIRLengthsIn.Value;

== matlab function Model_TranslationEngine64/ModelPreAmp/DecRate/Medusa5H1/MedusaHoligram/Medusa5H1 Part 6/Speaker Delay Tune/Output Delay Translation with Headrest/translation ==
  data: tuneNonHRDelaySamples input; tuneHRDrvDelaySamples input; tuneHRPaxDelaySamples input; tuneFREQDelaySamples input; DRDelay output; FRSpkrDelay output; DecimationFactor parameter; maxFullRateHoligramDelay parameter; maxFullRateSpeakerDelay parameter; numHeadrestComps parameter
  events: trigger input FUNCTION_CALL_EVENT
function [DRDelay, FRSpkrDelay] = fcn( tuneNonHRDelaySamples, tuneHRDrvDelaySamples, ...
    tuneHRPaxDelaySamples, tuneFREQDelaySamples, DecimationFactor, maxFullRateHoligramDelay, maxFullRateSpeakerDelay, numHeadrestComps)
%#codegen
%[Param:DecimationFactor]
%[Param:maxFullRateHoligramDelay]
%[Param:maxFullRateSpeakerDelay]
%[Param:numHeadrestComps]

nonHRDelaySamples = tuneNonHRDelaySamples.Value;
HRDrvDelaySamples = tuneHRDrvDelaySamples.Value;
HRPaxDelaySamples = tuneHRPaxDelaySamples.Value;
FREQDelaySamples = int32(tuneFREQDelaySamples.Value);

% Get delay upper bounds
maxFREQDelay = maxFullRateHoligramDelay;
maxFRSpkrDelay = maxFullRateSpeakerDelay;

% Compute delay values in samples
DEC = DecimationFactor;
% sampleRate = sampleRate;
FRHRDrvDelaySamples = round(HRDrvDelaySamples);
FRHRPaxDelaySamples = round(HRPaxDelaySamples);
FRNonHRDelaySamples = round(nonHRDelaySamples);

% Check whether speaker delays are multiple of 4, and if not round them up 
% to the nearest multiple
rem = ceil(FRNonHRDelaySamples/4)*4 - FRNonHRDelaySamples;
FRNonHRDelaySamples = int32(FRNonHRDelaySamples + rem);
DRNonHRDelaySamples = int32(FRNonHRDelaySamples/DEC);
if any(rem ~= 0)
    TranslateError('Speaker delays must be a multiple of 4.');
end

rem = ceil(FRHRDrvDelaySamples/4)*4 - FRHRDrvDelaySamples;
FRHRDrvDelaySamples = int32(FRHRDrvDelaySamples + rem);
DRHRDrvDelaySamples = int32(FRHRDrvDelaySamples/DEC);
if any(rem ~= 0)
    TranslateError('Driver headrest speaker delay must be a multiple of 4.');
end

rem = ceil(FRHRPaxDelaySamples/4)*4 - FRHRPaxDelaySamples;
FRHRPaxDelaySamples = int32(FRHRPaxDelaySamples + rem);
DRHRPaxDelaySamples = int32(FRHRPaxDelaySamples/DEC);
if any(rem ~= 0)
    TranslateError('Passenger headrest speaker delay must be a multiple of 4.');
end

% Check if delays are within bounds
checkDelay(FREQDelaySamples, maxFREQDelay, 'Medusa HFEQ delay');
checkDelay(FRHRDrvDelaySamples, maxFRSpkrDelay, 'h01/h0r delay');
checkDelay(FRHRPaxDelaySamples, maxFRSpkrDelay, 'h1l/h1r delay');
checkDelay(FRNonHRDelaySamples, maxFRSpkrDelay, 'Medusa non-headrest speaker delay');

% Assign values to TOPs
HRcomps = int32(ones(1,numHeadrestComps));
HRDrvDelay = DRHRDrvDelaySamples * HRcomps;
HRPaxDelay = DRHRPaxDelaySamples * HRcomps;
DRDelay = [DRNonHRDelaySamples, HRDrvDelay, HRPaxDelay];
FRSpkrDelay = FREQDelaySamples + [FRNonHRDelaySamples, FRHRDrvDelaySamples, ...
    FRHRPaxDelaySamples, FRHRDrvDelaySamples, FRHRPaxDelaySamples];
end


function checkDelay(delayValue, upper, name)

% Check if delays are within bounds
if(sum(delayValue < 0))
    TranslateError('Value of %s must be greater than or equal to zero.', name);
end

if(sum(delayValue > upper))
    TranslateError('Value of %s must be less than or equal to %d.', name, upper);
end

end

== matlab function Model_TranslationEngine64/InputSelect/Router/Trivial Translation ==
  data: OutMap output; Map input; nInRouterMask parameter
  events: trigger input FUNCTION_CALL_EVENT
function OutMap  = fcn(Map, nInRouterMask)
%#codegen

% ----- To access TuneVar maximum size, current size, and current value:
%   Note: TuneVar signals arrive with exposed variable size information.
%         The expressions below illustrate for the "Map" input argument.
%
%   size(Map.Value) : the maximum possible size of the Map variable
%
%   Tune.Size   : the current size of *valid* data in Map.Value
%
%   Map.Size(1) : Number of rows present in Map - this does not vary.
%
%   Map.Size(2) : Number of columns currently valid in Map - this is
%       the variable part of size that can change (if allowed by TuneVar).
%
%   Map.Value : the current value of the tune variable... but end-padded 
%       to the maximum available size with undefined/invalid data.
%
%   numel(Map.Value) : another way of looking at the maximum number of
%       elements that could arrive in Map.Value
%
% ----- To register an error, use the following method (works like printf):
%   TranslateError( <format string>, <arguments ... )
%   ... this error will cause the build process to abort.


% The below logic ensures that an output map gets filled in in the 
% "round robin" manner. This is to occur when the supplied map is shorter
% than the number of channel outputs. For instance,
% nChanIn = 4
% nChanOut = 9
% outputMapSupplied = [4 3 2 2]
% 
% This logic would run and return OutMap = [4 3 2 2 1 2 3 4 1]
%
% If no outputMap was supplied (i.e. = [];) THEN
% This logic would run and return OutMap = [1 2 3 4 1 2 3 4 1];


% First part finds the number of output map indices that were left blank
nChanOut = numel(Map.Value);
mapLength = Map.Size(2);
mapDifference = nChanOut - mapLength;
OutMap = int32(Map.Value);

% This loop appropriates the correct input channel number to the
% corresponding output channel, based on the mapDifference found above
if (mapLength == 1) && Map.Value(1) == 0
    mapLength = 0;
    mapDifference = nChanOut;
end
endOfMap = 0;
loopCount = 0;
while endOfMap < mapDifference
    for inputChan = 1 : nInRouterMask
        OutMap(mapLength+inputChan+loopCount) = inputChan;
        endOfMap = endOfMap + 1;
        if endOfMap == mapDifference
            break
        end
    end
    inputChan = 1;
    loopCount = loopCount + nInRouterMask;
end
